simulink model "blink_exec"  (Simulink 3.00)
libraries: execlib x6

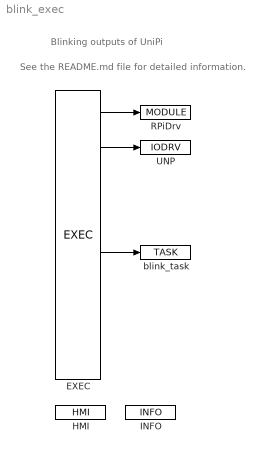
== system blink_exec ==
  note: See the README.md file for detailed information.
  note: Blinking outputs of UniPi
  EXEC : execlib/EXEC  target=Generic target device  tick=0.02  ntick0=1  ntick1=50  ntick2=100  ntick3=1200  pri0=5  pri1=9  pri2=13  pri3=18
  HMI : execlib/HMI  IncludeHMI=on  HmiDir=hmi  SourceDir=hmisrc  GenerateWebWatch=on  GenerateRexHMI=on  RedirectToHMI=off  Compression=off
  INFO : execlib/INFO  Title=UniPi - Blink example  Author=REX Controls s.r.o.  Description="UniPi - \"Hello world\""  Customer=Users of the REX Control System
  RPiDrv : execlib/MODULE
  UNP : execlib/IODRV  module=RPiDrv  classname=UnpDrv  factor=1  stack=10240  pri=3  timer=off
  blink_task : execlib/TASK  factor=1  start=0  stop=1  stack=10240  MDLOPEN=on
  wires:
  EXEC/1 -> RPiDrv/1
  EXEC/2 -> UNP/1
  EXEC/5 -> blink_task/1
